simulink model "buildiing_model"  (R2023a)
settings: Solver=VariableStepAuto  StartTime=0.0  StopTime=10.0  RelTol=1e-3
settings Model: Creator=NADJICH  LastModifiedBy=NADJICH

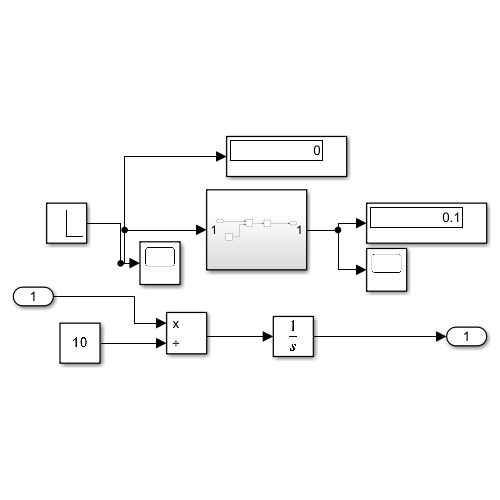
[thumbnail: Simulink's stored preview of the top-level diagram]
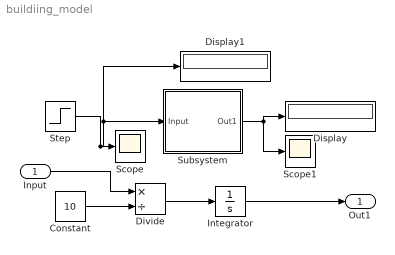
== system buildiing_model ==
  Input : Inport
  Constant : Constant  Value=10
  Display : Display
  Display1 : Display
  Divide : Product  Inputs=*/
  Integrator : Integrator
  Scope : Scope
  Scope1 : Scope
  Step : Step  Before=1  After=0  SampleTime=0
  Subsystem : Subsystem
  Out1 : Outport
  wires:
  Step/1 -> Scope/1, Display1/1, Subsystem/1(Input)
  Subsystem/1(Out1) -> Display/1, Scope1/1
  Integrator/1 -> Out1/1
  Input/1 -> Divide/1
  Divide/1 -> Integrator/1
  Constant/1 -> Divide/2

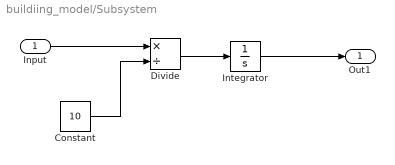
== system buildiing_model/Subsystem ==
  Input : Inport
  Constant : Constant  Value=10
  Divide : Product  Inputs=*/
  Integrator : Integrator
  Out1 : Outport
  wires:
  Integrator/1 -> Out1/1
  Input/1 -> Divide/1
  Divide/1 -> Integrator/1
  Constant/1 -> Divide/2
